simulink model "alphabetaPLL_test_sequence"  (R2020b)
settings: Solver=FixedStepAuto  StartTime=0.0  StopTime=40.6  FixedStep=1e-5
undefined symbols (not defined in the file or in its folder): f_rad
libraries: bach_library x2, simulink x1
settings Model: Creator=martin  LastModifiedBy=Kasper Laustsen
settings DataIOCC: ExternalInput=tt1, tt2, tt3, tt4, tt5, tt6  LoadExternalInput=on

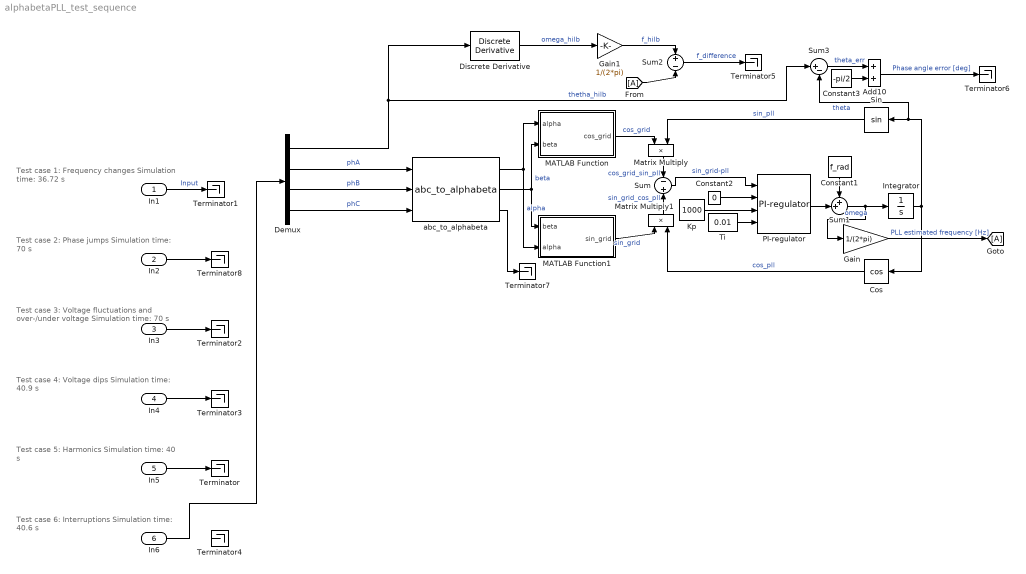
== system alphabetaPLL_test_sequence ==
  note: Test case 2: Phase jumps
      | Simulation time: 70 s
  note: Test case 1: Frequency changes
      | Simulation time: 36.72 s
  note: Test case 3: Voltage fluctuations
      | and over-/under voltage
      | Simulation time: 70 s
  note: Test case 4: Voltage dips
      | Simulation time: 40.9 s
  note: Test case 5: Harmonics
      | Simulation time: 40 s
  note: Test case 6: Interruptions
      | Simulation time: 40.6 s
  In1 : Inport  PortDimensions=4
  In2 : Inport  Port=2  PortDimensions=4
  In3 : Inport  Port=3  PortDimensions=4
  In4 : Inport  Port=4  PortDimensions=4
  In5 : Inport  Port=5  PortDimensions=4
  In6 : Inport  Port=6  PortDimensions=4
  Add10 : Sum
  Constant1 : Constant  Value=f_rad
  Constant2 : Constant  Value=0
  Constant3 : Constant  Value=-pi/2
  Cos : Trigonometry  Operator=cos
  Demux : Demux
  Discrete Derivative : simulink/Discrete/Discrete Derivative  gainval=1.0  ICPrevScaledInput=0.0  OutMin=[]  OutMax=[]  OutDataType=fixdt(1, 16)  OutScaling=2^-10  DoSatur=off
  Gain : Gain  Gain=1/(2*pi)
  Gain1 : Gain  Gain=1/(2*pi)
  Integrator : Integrator  IgnoreLimit=on
  Kp : Constant  Value=1000
  MATLAB Function : MATLAB Function  TreatAsAtomicUnit=on
  MATLAB Function1 : MATLAB Function  TreatAsAtomicUnit=on
  Matrix Multiply : Product
  Matrix Multiply1 : Product
  PI-regulator : bach_library/PI-regulator  SystemSampleTime=-1  VariantActivationTime=update diagram  Latency=0  AutoFrameSizeCalculation=off
  Sin : Trigonometry
  Sum : Sum  Inputs=-|+
  Sum1 : Sum  Inputs=++|
  Sum2 : Sum  Inputs=+|-
  Sum3 : Sum  Inputs=|+-
  Terminator{,1..8} (9 alike) : Terminator
  Ti : Constant  Value=0.01
  abc_to_alphabeta : bach_library/abc_to_alphabeta  SystemSampleTime=-1  VariantActivationTime=update diagram  Latency=0  AutoFrameSizeCalculation=off
  wires:
  abc_to_alphabeta/1 -> MATLAB Function/1(alpha), MATLAB Function1/2(alpha)  "alpha"
  abc_to_alphabeta/2 -> MATLAB Function/2(beta), MATLAB Function1/1(beta)  "beta"
  Matrix Multiply1/1 -> Sum/2  "sin_grid_cos_pll"
  Matrix Multiply/1 -> Sum/1  "cos_grid_sin_pll"
  Ti/1 -> PI-regulator/4
  Kp/1 -> PI-regulator/3
  Sum/1 -> PI-regulator/1  "sin_grid-pll"
  Constant2/1 -> PI-regulator/2
  PI-regulator/1 -> Sum1/2
  Constant1/1 -> Sum1/1
  Sum1/1 -> Gain/1, Integrator/1  "omega"
  Sin/1 -> Matrix Multiply/2  "sin_pll"
  Cos/1 -> Matrix Multiply1/2  "cos_pll"
  MATLAB Function1/1(sin_grid) -> Matrix Multiply1/1  "sin_grid"
  MATLAB Function/1(cos_grid) -> Matrix Multiply/1  "cos_grid"
  In1/1 -> Terminator1/1  "Input"
  Demux/2 -> abc_to_alphabeta/1  "phA"
  Demux/3 -> abc_to_alphabeta/2  "phB"
  In2/1 -> Terminator8/1
  In3/1 -> Terminator2/1
  In4/1 -> Terminator3/1
  In5/1 -> Terminator/1
  In6/1 -> Demux/1
  Gain/1 -> [A]  "PLL estimated frequency [Hz]"
  Demux/4 -> abc_to_alphabeta/3  "phC"
  Add10/1 -> Terminator6/1  "Phase angle error [deg]"
  Sum3/1 -> Add10/1  "theta_err"
  Constant3/1 -> Add10/2
  Integrator/1 -> Cos/1, Sum3/2, Sin/1  "theta"
  Demux/1 -> Discrete Derivative/1, Sum3/1  "thetha_hilb"
  abc_to_alphabeta/3 -> Terminator7/1
  Discrete Derivative/1 -> Gain1/1  "omega_hilb"
  Gain1/1 -> Sum2/1  "f_hilb"
  [A] -> Sum2/2
  Sum2/1 -> Terminator5/1  "f_difference"

== matlab function alphabetaPLL_test_sequence/MATLAB Function ==
  data: alpha input; cos_grid output; beta input
function cos_grid = cos_grid(alpha, beta)

cos_grid = alpha/sqrt(alpha^2+beta^2);

== matlab function alphabetaPLL_test_sequence/MATLAB Function1 ==
  data: beta input; alpha input; sin_grid output
function sin_grid = sin_grid(beta, alpha)

sin_grid = beta/sqrt(alpha^2+beta^2);
